simulink subsystem "ComputeIfChanged2"  (R2024a)
settings: Solver=VariableStepAuto  StartTime=0.0  StopTime=10.0  RelTol=1e-3
settings Model: Creator=dfurodet  LastModifiedBy=dfurodet

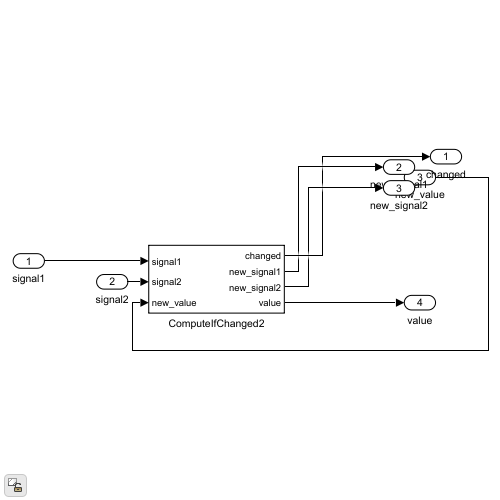
[thumbnail: Simulink's stored preview of the top-level diagram]
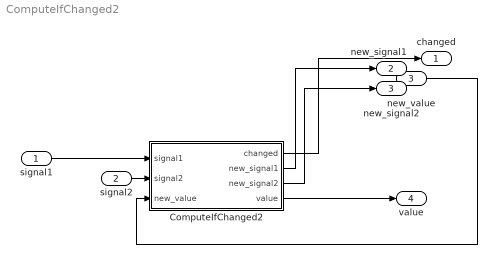
== system ComputeIfChanged2 ==
  signal1 : Inport
  signal2 : Inport  Port=2
  new_value : Inport  Port=3
  ComputeIfChanged2 : Subsystem
  changed : Outport
  new_signal1 : Outport  Port=2
  new_signal2 : Outport  Port=3
  value : Outport  Port=4
  wires:
  ComputeIfChanged2/1(changed) -> changed/1
  ComputeIfChanged2/3(new_signal2) -> new_signal2/1
  ComputeIfChanged2/2(new_signal1) -> new_signal1/1
  ComputeIfChanged2/4(value) -> value/1
  signal2/1 -> ComputeIfChanged2/2(signal2)
  signal1/1 -> ComputeIfChanged2/1(signal1)
  new_value/1 -> ComputeIfChanged2/3(new_value)

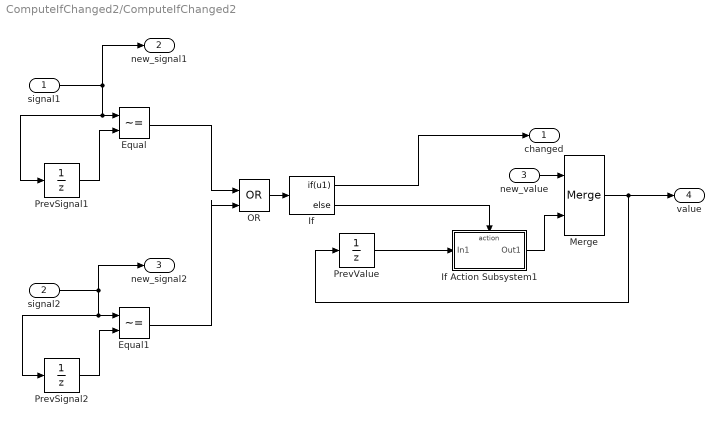
== system ComputeIfChanged2/ComputeIfChanged2 ==
  signal1 : Inport
  signal2 : Inport  Port=2
  new_value : Inport  Port=3
  Equal : RelationalOperator  Operator=~=  OutDataTypeStr=boolean  RndMeth=Simplest  InputSameDT=off
  Equal1 : RelationalOperator  Operator=~=  OutDataTypeStr=boolean  RndMeth=Simplest  InputSameDT=off
  If : If  IfExpression=u1
  If Action Subsystem1 : Subsystem  TreatAsAtomicUnit=on
  Merge : Merge
  OR : Logic  Operator=OR  IconShape=distinctive  AllPortsSameDT=off  OutDataTypeStr=boolean
  PrevSignal1 : UnitDelay  SampleTime=-1  HasFrameUpgradeWarning=on
  PrevSignal2 : UnitDelay  SampleTime=-1  HasFrameUpgradeWarning=on
  PrevValue : UnitDelay  SampleTime=-1  HasFrameUpgradeWarning=on
  changed : Outport
  new_signal1 : Outport  Port=2
  new_signal2 : Outport  Port=3
  value : Outport  Port=4
  wires:
  Equal/1 -> OR/1
  OR/1 -> If/1
  Equal1/1 -> OR/2
  PrevSignal2/1 -> Equal1/2
  signal2/1 -> new_signal2/1, Equal1/1, PrevSignal2/1
  PrevValue/1 -> If Action Subsystem1/1(In1)
  If Action Subsystem1/1(Out1) -> Merge/2
  new_value/1 -> Merge/1
  PrevSignal1/1 -> Equal/2
  If/2 -> If Action Subsystem1/Action
  signal1/1 -> PrevSignal1/1, Equal/1, new_signal1/1
  If/1 -> changed/1
  Merge/1 -> PrevValue/1, value/1

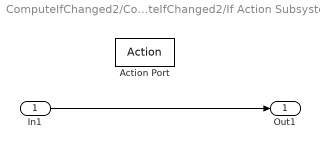
== system ComputeIfChanged2/ComputeIfChanged2/If Action Subsystem1 ==
  In1 : Inport
  Action Port : ActionPort
  Out1 : Outport
  wires:
  In1/1 -> Out1/1
